simulink subsystem "First_simul_model"  (R2021b)
settings: Solver=VariableStepAuto  StartTime=0.0  StopTime=10.0  RelTol=1e-3
settings Model: Creator=adana  LastModifiedBy=adana

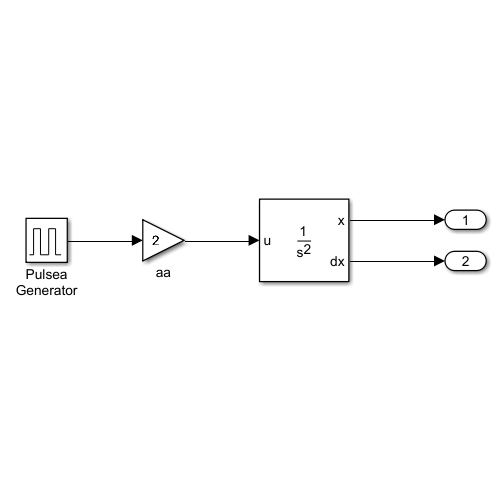
[thumbnail: Simulink's stored preview of the top-level diagram]
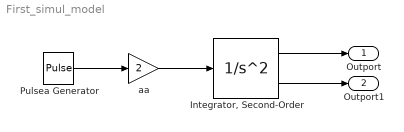
== system First_simul_model ==
  "Integrator, Second-Order" : SecondOrderIntegrator
  Pulsea Generator : DiscretePulseGenerator  PulseType=Time based  Period=10  PulseWidth=5
  aa : Gain  Gain=2
  Outport : Outport
  Outport1 : Outport  Port=2
  wires:
  Pulsea Generator/1 -> aa/1
  aa/1 -> "Integrator, Second-Order"/1
  "Integrator, Second-Order"/1 -> Outport/1
  "Integrator, Second-Order"/2 -> Outport1/1
